simulink library "mech_robot_vrlib"  (Simulink 6.0)
settings: Solver=ode45  SolverMode=SingleTasking  StartTime=0.0  StopTime=10.0  RelTol=1e-3
libraries: vrlib x1
settings Model: Creator=arnav  LastModifiedBy=batserve  ExtModeAutoUpdateStatusClock=off
settings OptimizationCC: BooleanDataType=off
settings DebuggingCC: SolverPrmCheckMsg=none
settings HardwareCC: TargetUnknown=on

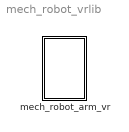
== system mech_robot_vrlib ==
  mech_robot_arm_vr : Subsystem

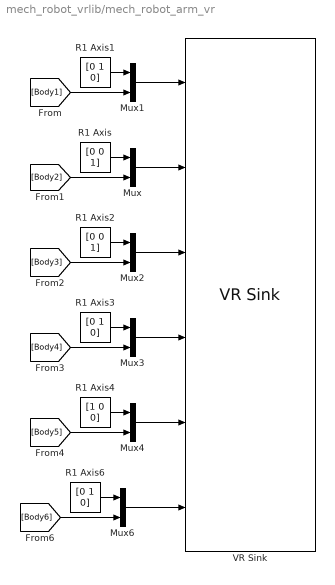
== system mech_robot_vrlib/mech_robot_arm_vr ==
  Mux{,1..4,6} (6 alike) : Mux  Inputs=2
  R1 Axis : Constant  Value=[0 0 1]
  R1 Axis1 : Constant  Value=[0 1 0]
  R1 Axis2 : Constant  Value=[0 0 1]
  R1 Axis3 : Constant  Value=[0 1 0]
  R1 Axis4 : Constant  Value=[1 0 0]
  R1 Axis6 : Constant  Value=[0 1 0]
  VR Sink : vrlib/VR Sink  SampleTime=0.01  ViewEnable=on  RemoteChange=off  RemoteView=off  FieldsWritten=rbody1.rotation.4#rbody2.rotation.4#rbody3.rotation.4#rbody4.rotation.4#rbody5.rotation.4#drill.rotation.4  WorldFileName=robotamain.wrl  WorldDescription=robotamain  AutoView=off  FigureProperties={'Position', 'Name', 'Viewpoint', 'CameraBound', 'CameraDirection', 'CameraPosition', 'CameraUpVector', 'ZoomFactor', 'Antialiasing', 'Headlight', 'Lighting', 'PanelMode', 'Textures', 'Transparency', 'Wireframe', 'DeleteFcn', ; }
      settings: AttributesFormatString=\n\n\n\n\n\n
  wires:
  Mux4/1 -> VR Sink/5
  Mux3/1 -> VR Sink/4
  Mux2/1 -> VR Sink/3
  Mux/1 -> VR Sink/2
  Mux1/1 -> VR Sink/1
  Mux6/1 -> VR Sink/6
  [Body6] -> Mux6/2
  R1 Axis6/1 -> Mux6/1
  [Body5] -> Mux4/2
  [Body4] -> Mux3/2
  [Body3] -> Mux2/2
  [Body2] -> Mux/2
  [Body1] -> Mux1/2
  R1 Axis4/1 -> Mux4/1
  R1 Axis3/1 -> Mux3/1
  R1 Axis2/1 -> Mux2/1
  R1 Axis1/1 -> Mux1/1
  R1 Axis/1 -> Mux/1
